simulink model "l64_dev"  (Simulink 7.9)
settings: Solver=ode45  StartTime=0.0  StopTime=525000  RelTol=1e-3
undefined symbols (not defined in the file): sfp
libraries: xbsIndex_r4 x835, xps_library x23, casper_library_delays x22, casper_library_misc x3
(part 3 of 8)

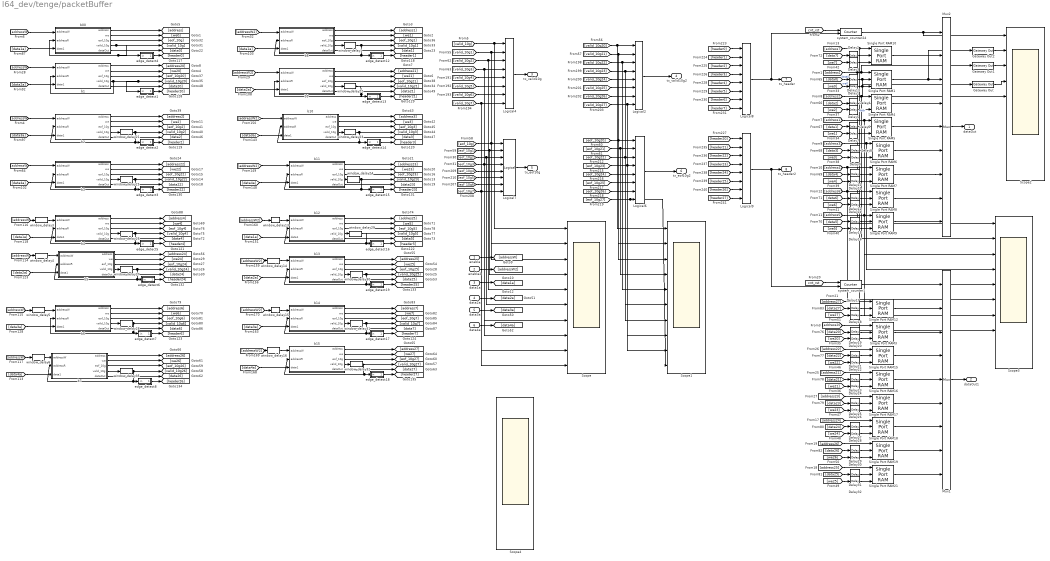
== system l64_dev/tenge/packetBuffer ==
  enable : Inport
  enable2 : Inport  Port=2
  data1a : Inport  Port=3
  data2a : Inport  Port=4
  data3a : Inport  Port=5
  data4a : Inport  Port=6
  Delay{1..32} (32 alike) : xbsIndex_r4/Delay  rst=off  infoeditControl=Selection of Reset will increase slice count due to use of real FFs and instead of SRLs  en=off  latency=2  dbl_ovrd=off  reg_retiming=on  block_type=delay
      settings: xl_area=[0, 0, 0, 0, 0, 0, 0]
  Gateway Out : xbsIndex_r4/Gateway Out  inherit_from_input=off  hdl_port=on  timing_constraint=None  locs_specified=off  LOCs={}  UseAsDAC=off  DACChannel='1'  block_type=gatewayout
  Gateway Out1 : xbsIndex_r4/Gateway Out  inherit_from_input=off  hdl_port=on  timing_constraint=None  locs_specified=off  LOCs={}  UseAsDAC=off  DACChannel='1'  block_type=gatewayout
  Gateway Out2 : xbsIndex_r4/Gateway Out  inherit_from_input=off  hdl_port=on  timing_constraint=None  locs_specified=off  LOCs={}  UseAsDAC=off  DACChannel='1'  block_type=gatewayout
  Logical{2,4,6..7} (4 alike) : xbsIndex_r4/Logical  logical_function=OR  inputs=8  en=off  latency=8  precision=Full  arith_type=Unsigned  n_bits=16  bin_pt=0  align_bp=on  dbl_ovrd=off  block_type=logical
      settings: block_version=11.4
  Logical8 : xbsIndex_r4/Logical  logical_function=OR  inputs=8  en=off  latency=4  precision=Full  arith_type=Unsigned  n_bits=16  bin_pt=0  align_bp=on  dbl_ovrd=off  block_type=logical
      settings: block_version=11.4
  Logical9 : xbsIndex_r4/Logical  logical_function=OR  inputs=8  en=off  latency=4  precision=Full  arith_type=Unsigned  n_bits=16  bin_pt=0  align_bp=on  dbl_ovrd=off  block_type=logical
      settings: block_version=11.4
  Mux1 : xbsIndex_r4/Mux  inputs=8  en=off  latency=2  precision=Full  arith_type="Signed  (2's comp)"  n_bits=8  bin_pt=2  quantization=Truncate  overflow=Wrap  dbl_ovrd=off  block_type=mux
      settings: xl_area=[0, 0, 0, 0, 0, 0, 0]
  Mux2 : xbsIndex_r4/Mux  inputs=8  en=off  latency=2  precision=Full  arith_type="Signed  (2's comp)"  n_bits=8  bin_pt=2  quantization=Truncate  overflow=Wrap  dbl_ovrd=off  block_type=mux
      settings: xl_area=[0, 0, 0, 0, 0, 0, 0]
  Scope{,1..4} (5 alike) : Scope  NumInputPorts=10
      Scope settings: YMin=0~0~0~4012~3800.95~-1~-5~-5~-5~-5  YMax=7000~1~1~4022~4201.05~1~5~5~5~5  SaveName=ScopeData3
      Scope1 settings: YMin=0~0~0~4012~3800.95~-1~-5~-5~-5~-5  YMax=7000~1~1~4022~4201.05~1~5~5~5~5  SaveName=ScopeData4
      Scope2 settings: YMin=0~0~0~4012~3800.95~-1~-5~-5~-5~-5  YMax=7000~1~1~4022~4201.05~1~5~5~5~5  SaveName=ScopeData5
      Scope3 settings: YMin=0~0~0~4012~3800.95~-1~-5~-5~-5~-5  YMax=7000~1~1~4022~4201.05~1~5~5~5~5  SaveName=ScopeData14
      Scope4 settings: YMin=0~0~0~4012~3800.95~-1~-5~-5~-5~-5  YMax=7000~1~1~4022~4201.05~1~5~5~5~5  SaveName=ScopeData16
  Single Port RAM{1,3..10,12,15..19,21} (16 alike) : xbsIndex_r4/Single Port RAM  depth=872  initVector=0  distributed_mem=Block RAM  write_mode=No Read On Write  rst=off  init_reg=0  en=off  latency=4  dbl_ovrd=off  optimize=Area  use_rpm=on  block_type=spram
  b00 : Subsystem
  b1 : Subsystem
  b10 : Subsystem
  b11 : Subsystem
  b12 : Subsystem
  b13 : Subsystem
  b14 : Subsystem
  b15 : Subsystem
  b2 : Subsystem
  b3 : Subsystem
  b4 : Subsystem
  b5 : Subsystem
  b6 : Subsystem
  b7 : Subsystem
  b8 : Subsystem
  b9 : Subsystem
  edge_detect1 : Subsystem  AncestorBlock=casper_library_misc/edge_detect  mask(edge_detect){edge=Rising, polarity=Active High, x_in=[0 0.08 0.08 0.16 0.16 0.24 0.24 0.32 0.32 0.4], y_in=[-1 -1  1  1  1  1  1  1  1  1], x_out=[0.6 0.68 0.68 0.76 0.76 0.84 0.84 0.92 0.92 1], y_out=[-1 -1  1  1 -1 -1 -1 -1 -1 -1]}
      mask prompts: edge "Edge Type"; polarity "Output Polarity"; x_in "Input X Positions"; y_in "Input Y Positions"; x_out "Output X Positions"; y_out "Output Y Positions"
      mask help: Output is active for one-cycle after each edge of the specified type (i.e. rising, falling or both).
      mask init: same as l64_dev/misc/edge_detect1
      settings: AttributesFormatString=|
      | rising edges
      | active high
      mask Help: Output is active for one-cycle after each edge of the specified type (i.e. rising, falling, or both).  Latency is zero.
      mask StyleString: popup(Rising|Falling|Both),popup(Active High|Active Low),edit,edit,edit,edit
      mask Display:
      | plot(x_in_num,0.5+y_in_num*0.2);
      | plot(x_out_num,0.5+y_out_num*0.2);
  edge_detect12 : Subsystem  AncestorBlock=casper_library_misc/edge_detect  mask(edge_detect){edge=Rising, polarity=Active High, x_in=[0 0.08 0.08 0.16 0.16 0.24 0.24 0.32 0.32 0.4], y_in=[-1 -1  1  1  1  1  1  1  1  1], x_out=[0.6 0.68 0.68 0.76 0.76 0.84 0.84 0.92 0.92 1], y_out=[-1 -1  1  1 -1 -1 -1 -1 -1 -1]}
      mask prompts: edge "Edge Type"; polarity "Output Polarity"; x_in "Input X Positions"; y_in "Input Y Positions"; x_out "Output X Positions"; y_out "Output Y Positions"
      mask help: Output is active for one-cycle after each edge of the specified type (i.e. rising, falling or both).
      mask init: same as l64_dev/misc/edge_detect1
      settings: AttributesFormatString=|
      | rising edges
      | active high
      mask Help: Output is active for one-cycle after each edge of the specified type (i.e. rising, falling, or both).  Latency is zero.
      mask StyleString: popup(Rising|Falling|Both),popup(Active High|Active Low),edit,edit,edit,edit
      mask Display:
      | plot(x_in_num,0.5+y_in_num*0.2);
      | plot(x_out_num,0.5+y_out_num*0.2);
  edge_detect13 : Subsystem  AncestorBlock=casper_library_misc/edge_detect  mask(edge_detect){edge=Rising, polarity=Active High, x_in=[0 0.08 0.08 0.16 0.16 0.24 0.24 0.32 0.32 0.4], y_in=[-1 -1  1  1  1  1  1  1  1  1], x_out=[0.6 0.68 0.68 0.76 0.76 0.84 0.84 0.92 0.92 1], y_out=[-1 -1  1  1 -1 -1 -1 -1 -1 -1]}
      mask prompts: edge "Edge Type"; polarity "Output Polarity"; x_in "Input X Positions"; y_in "Input Y Positions"; x_out "Output X Positions"; y_out "Output Y Positions"
      mask help: Output is active for one-cycle after each edge of the specified type (i.e. rising, falling or both).
      mask init: same as l64_dev/misc/edge_detect1
      settings: AttributesFormatString=|
      | rising edges
      | active high
      mask Help: Output is active for one-cycle after each edge of the specified type (i.e. rising, falling, or both).  Latency is zero.
      mask StyleString: popup(Rising|Falling|Both),popup(Active High|Active Low),edit,edit,edit,edit
      mask Display:
      | plot(x_in_num,0.5+y_in_num*0.2);
      | plot(x_out_num,0.5+y_out_num*0.2);
  edge_detect14 : Subsystem  AncestorBlock=casper_library_misc/edge_detect  mask(edge_detect){edge=Rising, polarity=Active High, x_in=[0 0.08 0.08 0.16 0.16 0.24 0.24 0.32 0.32 0.4], y_in=[-1 -1  1  1  1  1  1  1  1  1], x_out=[0.6 0.68 0.68 0.76 0.76 0.84 0.84 0.92 0.92 1], y_out=[-1 -1  1  1 -1 -1 -1 -1 -1 -1]}
      mask prompts: edge "Edge Type"; polarity "Output Polarity"; x_in "Input X Positions"; y_in "Input Y Positions"; x_out "Output X Positions"; y_out "Output Y Positions"
      mask help: Output is active for one-cycle after each edge of the specified type (i.e. rising, falling or both).
      mask init: same as l64_dev/misc/edge_detect1
      settings: AttributesFormatString=|
      | rising edges
      | active high
      mask Help: Output is active for one-cycle after each edge of the specified type (i.e. rising, falling, or both).  Latency is zero.
      mask StyleString: popup(Rising|Falling|Both),popup(Active High|Active Low),edit,edit,edit,edit
      mask Display:
      | plot(x_in_num,0.5+y_in_num*0.2);
      | plot(x_out_num,0.5+y_out_num*0.2);
  edge_detect15 : Subsystem  AncestorBlock=casper_library_misc/edge_detect  mask(edge_detect){edge=Rising, polarity=Active High, x_in=[0 0.08 0.08 0.16 0.16 0.24 0.24 0.32 0.32 0.4], y_in=[-1 -1  1  1  1  1  1  1  1  1], x_out=[0.6 0.68 0.68 0.76 0.76 0.84 0.84 0.92 0.92 1], y_out=[-1 -1  1  1 -1 -1 -1 -1 -1 -1]}
      mask prompts: edge "Edge Type"; polarity "Output Polarity"; x_in "Input X Positions"; y_in "Input Y Positions"; x_out "Output X Positions"; y_out "Output Y Positions"
      mask help: Output is active for one-cycle after each edge of the specified type (i.e. rising, falling or both).
      mask init: same as l64_dev/misc/edge_detect1
      settings: AttributesFormatString=|
      | rising edges
      | active high
      mask Help: Output is active for one-cycle after each edge of the specified type (i.e. rising, falling, or both).  Latency is zero.
      mask StyleString: popup(Rising|Falling|Both),popup(Active High|Active Low),edit,edit,edit,edit
      mask Display:
      | plot(x_in_num,0.5+y_in_num*0.2);
      | plot(x_out_num,0.5+y_out_num*0.2);
  edge_detect16 : Subsystem  AncestorBlock=casper_library_misc/edge_detect  mask(edge_detect){edge=Rising, polarity=Active High, x_in=[0 0.08 0.08 0.16 0.16 0.24 0.24 0.32 0.32 0.4], y_in=[-1 -1  1  1  1  1  1  1  1  1], x_out=[0.6 0.68 0.68 0.76 0.76 0.84 0.84 0.92 0.92 1], y_out=[-1 -1  1  1 -1 -1 -1 -1 -1 -1]}
      mask prompts: edge "Edge Type"; polarity "Output Polarity"; x_in "Input X Positions"; y_in "Input Y Positions"; x_out "Output X Positions"; y_out "Output Y Positions"
      mask help: Output is active for one-cycle after each edge of the specified type (i.e. rising, falling or both).
      mask init: same as l64_dev/misc/edge_detect1
      settings: AttributesFormatString=|
      | rising edges
      | active high
      mask Help: Output is active for one-cycle after each edge of the specified type (i.e. rising, falling, or both).  Latency is zero.
      mask StyleString: popup(Rising|Falling|Both),popup(Active High|Active Low),edit,edit,edit,edit
      mask Display:
      | plot(x_in_num,0.5+y_in_num*0.2);
      | plot(x_out_num,0.5+y_out_num*0.2);
  edge_detect17 : Subsystem  AncestorBlock=casper_library_misc/edge_detect  mask(edge_detect){edge=Rising, polarity=Active High, x_in=[0 0.08 0.08 0.16 0.16 0.24 0.24 0.32 0.32 0.4], y_in=[-1 -1  1  1  1  1  1  1  1  1], x_out=[0.6 0.68 0.68 0.76 0.76 0.84 0.84 0.92 0.92 1], y_out=[-1 -1  1  1 -1 -1 -1 -1 -1 -1]}
      mask prompts: edge "Edge Type"; polarity "Output Polarity"; x_in "Input X Positions"; y_in "Input Y Positions"; x_out "Output X Positions"; y_out "Output Y Positions"
      mask help: Output is active for one-cycle after each edge of the specified type (i.e. rising, falling or both).
      mask init: same as l64_dev/misc/edge_detect1
      settings: AttributesFormatString=|
      | rising edges
      | active high
      mask Help: Output is active for one-cycle after each edge of the specified type (i.e. rising, falling, or both).  Latency is zero.
      mask StyleString: popup(Rising|Falling|Both),popup(Active High|Active Low),edit,edit,edit,edit
      mask Display:
      | plot(x_in_num,0.5+y_in_num*0.2);
      | plot(x_out_num,0.5+y_out_num*0.2);
  edge_detect18 : Subsystem  AncestorBlock=casper_library_misc/edge_detect  mask(edge_detect){edge=Rising, polarity=Active High, x_in=[0 0.08 0.08 0.16 0.16 0.24 0.24 0.32 0.32 0.4], y_in=[-1 -1  1  1  1  1  1  1  1  1], x_out=[0.6 0.68 0.68 0.76 0.76 0.84 0.84 0.92 0.92 1], y_out=[-1 -1  1  1 -1 -1 -1 -1 -1 -1]}
      mask prompts: edge "Edge Type"; polarity "Output Polarity"; x_in "Input X Positions"; y_in "Input Y Positions"; x_out "Output X Positions"; y_out "Output Y Positions"
      mask help: Output is active for one-cycle after each edge of the specified type (i.e. rising, falling or both).
      mask init: same as l64_dev/misc/edge_detect1
      settings: AttributesFormatString=|
      | rising edges
      | active high
      mask Help: Output is active for one-cycle after each edge of the specified type (i.e. rising, falling, or both).  Latency is zero.
      mask StyleString: popup(Rising|Falling|Both),popup(Active High|Active Low),edit,edit,edit,edit
      mask Display:
      | plot(x_in_num,0.5+y_in_num*0.2);
      | plot(x_out_num,0.5+y_out_num*0.2);
  edge_detect19 : Subsystem  AncestorBlock=casper_library_misc/edge_detect  mask(edge_detect){edge=Rising, polarity=Active High, x_in=[0 0.08 0.08 0.16 0.16 0.24 0.24 0.32 0.32 0.4], y_in=[-1 -1  1  1  1  1  1  1  1  1], x_out=[0.6 0.68 0.68 0.76 0.76 0.84 0.84 0.92 0.92 1], y_out=[-1 -1  1  1 -1 -1 -1 -1 -1 -1]}
      mask prompts: edge "Edge Type"; polarity "Output Polarity"; x_in "Input X Positions"; y_in "Input Y Positions"; x_out "Output X Positions"; y_out "Output Y Positions"
      mask help: Output is active for one-cycle after each edge of the specified type (i.e. rising, falling or both).
      mask init: same as l64_dev/misc/edge_detect1
      settings: AttributesFormatString=|
      | rising edges
      | active high
      mask Help: Output is active for one-cycle after each edge of the specified type (i.e. rising, falling, or both).  Latency is zero.
      mask StyleString: popup(Rising|Falling|Both),popup(Active High|Active Low),edit,edit,edit,edit
      mask Display:
      | plot(x_in_num,0.5+y_in_num*0.2);
      | plot(x_out_num,0.5+y_out_num*0.2);
  edge_detect2 : Subsystem  AncestorBlock=casper_library_misc/edge_detect  mask(edge_detect){edge=Rising, polarity=Active High, x_in=[0 0.08 0.08 0.16 0.16 0.24 0.24 0.32 0.32 0.4], y_in=[-1 -1  1  1  1  1  1  1  1  1], x_out=[0.6 0.68 0.68 0.76 0.76 0.84 0.84 0.92 0.92 1], y_out=[-1 -1  1  1 -1 -1 -1 -1 -1 -1]}
      mask prompts: edge "Edge Type"; polarity "Output Polarity"; x_in "Input X Positions"; y_in "Input Y Positions"; x_out "Output X Positions"; y_out "Output Y Positions"
      mask help: Output is active for one-cycle after each edge of the specified type (i.e. rising, falling or both).
      mask init: same as l64_dev/misc/edge_detect1
      settings: AttributesFormatString=|
      | rising edges
      | active high
      mask Help: Output is active for one-cycle after each edge of the specified type (i.e. rising, falling, or both).  Latency is zero.
      mask StyleString: popup(Rising|Falling|Both),popup(Active High|Active Low),edit,edit,edit,edit
      mask Display:
      | plot(x_in_num,0.5+y_in_num*0.2);
      | plot(x_out_num,0.5+y_out_num*0.2);
  edge_detect3 : Subsystem  AncestorBlock=casper_library_misc/edge_detect  mask(edge_detect){edge=Rising, polarity=Active High, x_in=[0 0.08 0.08 0.16 0.16 0.24 0.24 0.32 0.32 0.4], y_in=[-1 -1  1  1  1  1  1  1  1  1], x_out=[0.6 0.68 0.68 0.76 0.76 0.84 0.84 0.92 0.92 1], y_out=[-1 -1  1  1 -1 -1 -1 -1 -1 -1]}
      mask prompts: edge "Edge Type"; polarity "Output Polarity"; x_in "Input X Positions"; y_in "Input Y Positions"; x_out "Output X Positions"; y_out "Output Y Positions"
      mask help: Output is active for one-cycle after each edge of the specified type (i.e. rising, falling or both).
      mask init: same as l64_dev/misc/edge_detect1
      settings: AttributesFormatString=|
      | rising edges
      | active high
      mask Help: Output is active for one-cycle after each edge of the specified type (i.e. rising, falling, or both).  Latency is zero.
      mask StyleString: popup(Rising|Falling|Both),popup(Active High|Active Low),edit,edit,edit,edit
      mask Display:
      | plot(x_in_num,0.5+y_in_num*0.2);
      | plot(x_out_num,0.5+y_out_num*0.2);
  edge_detect4 : Subsystem  AncestorBlock=casper_library_misc/edge_detect  mask(edge_detect){edge=Rising, polarity=Active High, x_in=[0 0.08 0.08 0.16 0.16 0.24 0.24 0.32 0.32 0.4], y_in=[-1 -1  1  1  1  1  1  1  1  1], x_out=[0.6 0.68 0.68 0.76 0.76 0.84 0.84 0.92 0.92 1], y_out=[-1 -1  1  1 -1 -1 -1 -1 -1 -1]}
      mask prompts: edge "Edge Type"; polarity "Output Polarity"; x_in "Input X Positions"; y_in "Input Y Positions"; x_out "Output X Positions"; y_out "Output Y Positions"
      mask help: Output is active for one-cycle after each edge of the specified type (i.e. rising, falling or both).
      mask init: same as l64_dev/misc/edge_detect1
      settings: AttributesFormatString=|
      | rising edges
      | active high
      mask Help: Output is active for one-cycle after each edge of the specified type (i.e. rising, falling, or both).  Latency is zero.
      mask StyleString: popup(Rising|Falling|Both),popup(Active High|Active Low),edit,edit,edit,edit
      mask Display:
      | plot(x_in_num,0.5+y_in_num*0.2);
      | plot(x_out_num,0.5+y_out_num*0.2);
  edge_detect5 : Subsystem  AncestorBlock=casper_library_misc/edge_detect  mask(edge_detect){edge=Rising, polarity=Active High, x_in=[0 0.08 0.08 0.16 0.16 0.24 0.24 0.32 0.32 0.4], y_in=[-1 -1  1  1  1  1  1  1  1  1], x_out=[0.6 0.68 0.68 0.76 0.76 0.84 0.84 0.92 0.92 1], y_out=[-1 -1  1  1 -1 -1 -1 -1 -1 -1]}
      mask prompts: edge "Edge Type"; polarity "Output Polarity"; x_in "Input X Positions"; y_in "Input Y Positions"; x_out "Output X Positions"; y_out "Output Y Positions"
      mask help: Output is active for one-cycle after each edge of the specified type (i.e. rising, falling or both).
      mask init: same as l64_dev/misc/edge_detect1
      settings: AttributesFormatString=|
      | rising edges
      | active high
      mask Help: Output is active for one-cycle after each edge of the specified type (i.e. rising, falling, or both).  Latency is zero.
      mask StyleString: popup(Rising|Falling|Both),popup(Active High|Active Low),edit,edit,edit,edit
      mask Display:
      | plot(x_in_num,0.5+y_in_num*0.2);
      | plot(x_out_num,0.5+y_out_num*0.2);
  edge_detect6 : Subsystem  AncestorBlock=casper_library_misc/edge_detect  mask(edge_detect){edge=Rising, polarity=Active High, x_in=[0 0.08 0.08 0.16 0.16 0.24 0.24 0.32 0.32 0.4], y_in=[-1 -1  1  1  1  1  1  1  1  1], x_out=[0.6 0.68 0.68 0.76 0.76 0.84 0.84 0.92 0.92 1], y_out=[-1 -1  1  1 -1 -1 -1 -1 -1 -1]}
      mask prompts: edge "Edge Type"; polarity "Output Polarity"; x_in "Input X Positions"; y_in "Input Y Positions"; x_out "Output X Positions"; y_out "Output Y Positions"
      mask help: Output is active for one-cycle after each edge of the specified type (i.e. rising, falling or both).
      mask init: same as l64_dev/misc/edge_detect1
      settings: AttributesFormatString=|
      | rising edges
      | active high
      mask Help: Output is active for one-cycle after each edge of the specified type (i.e. rising, falling, or both).  Latency is zero.
      mask StyleString: popup(Rising|Falling|Both),popup(Active High|Active Low),edit,edit,edit,edit
      mask Display:
      | plot(x_in_num,0.5+y_in_num*0.2);
      | plot(x_out_num,0.5+y_out_num*0.2);
  edge_detect7 : Subsystem  AncestorBlock=casper_library_misc/edge_detect  mask(edge_detect){edge=Rising, polarity=Active High, x_in=[0 0.08 0.08 0.16 0.16 0.24 0.24 0.32 0.32 0.4], y_in=[-1 -1  1  1  1  1  1  1  1  1], x_out=[0.6 0.68 0.68 0.76 0.76 0.84 0.84 0.92 0.92 1], y_out=[-1 -1  1  1 -1 -1 -1 -1 -1 -1]}
      mask prompts: edge "Edge Type"; polarity "Output Polarity"; x_in "Input X Positions"; y_in "Input Y Positions"; x_out "Output X Positions"; y_out "Output Y Positions"
      mask help: Output is active for one-cycle after each edge of the specified type (i.e. rising, falling or both).
      mask init: same as l64_dev/misc/edge_detect1
      settings: AttributesFormatString=|
      | rising edges
      | active high
      mask Help: Output is active for one-cycle after each edge of the specified type (i.e. rising, falling, or both).  Latency is zero.
      mask StyleString: popup(Rising|Falling|Both),popup(Active High|Active Low),edit,edit,edit,edit
      mask Display:
      | plot(x_in_num,0.5+y_in_num*0.2);
      | plot(x_out_num,0.5+y_out_num*0.2);
  edge_detect8 : Subsystem  AncestorBlock=casper_library_misc/edge_detect  mask(edge_detect){edge=Rising, polarity=Active High, x_in=[0 0.08 0.08 0.16 0.16 0.24 0.24 0.32 0.32 0.4], y_in=[-1 -1  1  1  1  1  1  1  1  1], x_out=[0.6 0.68 0.68 0.76 0.76 0.84 0.84 0.92 0.92 1], y_out=[-1 -1  1  1 -1 -1 -1 -1 -1 -1]}
      mask prompts: edge "Edge Type"; polarity "Output Polarity"; x_in "Input X Positions"; y_in "Input Y Positions"; x_out "Output X Positions"; y_out "Output Y Positions"
      mask help: Output is active for one-cycle after each edge of the specified type (i.e. rising, falling or both).
      mask init: same as l64_dev/misc/edge_detect1
      settings: AttributesFormatString=|
      | rising edges
      | active high
      mask Help: Output is active for one-cycle after each edge of the specified type (i.e. rising, falling, or both).  Latency is zero.
      mask StyleString: popup(Rising|Falling|Both),popup(Active High|Active Low),edit,edit,edit,edit
      mask Display:
      | plot(x_in_num,0.5+y_in_num*0.2);
      | plot(x_out_num,0.5+y_out_num*0.2);
  system_counter1 : xbsIndex_r4/Counter  cnt_type=Free Running  cnt_to=7  operation=Up  start_count=0  cnt_by_val=1  arith_type=Unsigned  n_bits=3  bin_pt=0  load_pin=off  rst=on  en=on  explicit_period=on  period=1  dbl_ovrd=off  use_behavioral_HDL=off  implementation=Fabric  block_type=counter
      settings: block_version=11.4
  system_counter24 : xbsIndex_r4/Counter  cnt_type=Free Running  cnt_to=7  operation=Up  start_count=0  cnt_by_val=1  arith_type=Unsigned  n_bits=3  bin_pt=0  load_pin=off  rst=on  en=on  explicit_period=on  period=1  dbl_ovrd=off  use_behavioral_HDL=off  implementation=Fabric  block_type=counter
      settings: block_version=11.4
  window_delay1 : casper_library_delays/window_delay  delay=1400
  window_delay{3..6,13..16} (8 alike) : casper_library_delays/window_delay  delay=1200
  window_delay21 : casper_library_delays/window_delay  delay=700
  window_delay22 : casper_library_delays/window_delay  delay=1400
  window_delay23 : casper_library_delays/window_delay  delay=2100
  window_delay24 : casper_library_delays/window_delay  delay=2100
  window_delay25 : casper_library_delays/window_delay  delay=700
  window_delay26 : casper_library_delays/window_delay  delay=2800
  window_delay27 : casper_library_delays/window_delay  delay=2800
  window_delay28 : casper_library_delays/window_delay  delay=3500
  window_delay29 : casper_library_delays/window_delay  delay=4200
  window_delay30 : casper_library_delays/window_delay  delay=4200
  window_delay31 : casper_library_delays/window_delay  delay=4900
  window_delay32 : casper_library_delays/window_delay  delay=4900
  window_delay35 : casper_library_delays/window_delay  delay=3500
  dataOut : Outport
  dataOut1 : Outport  Port=2
  tx_valid10g : Outport  Port=3
  tx_valid10g2 : Outport  Port=4
  tx_eof10g : Outport  Port=5
  tx_eof10g2 : Outport  Port=6
  tx_header : Outport  Port=7
  tx_header2 : Outport  Port=8
  wires:
  Single Port RAM1/1 -> Mux2/3, Gateway Out2/1
  Single Port RAM4/1 -> Mux2/4
  Single Port RAM5/1 -> Mux2/5
  Single Port RAM6/1 -> Mux2/6
  Single Port RAM7/1 -> Mux2/7
  Single Port RAM8/1 -> Mux2/8
  Mux2/1 -> dataOut/1
  Single Port RAM3/1 -> Mux1/3
  Single Port RAM15/1 -> Mux1/4
  Single Port RAM16/1 -> Mux1/5
  Single Port RAM17/1 -> Mux1/6
  Single Port RAM18/1 -> Mux1/7
  Single Port RAM19/1 -> Mux1/8
  Single Port RAM21/1 -> Mux1/9
  Mux1/1 -> dataOut1/1
  ? -> ?
  enable/1 -> [addressW]
  enable2/1 -> [addressW2]
  [addressW] -> b00/1(addressW)
  b00/1(address) -> [address]
  b00/2(we) -> [we0]
  [addressW] -> b1/1(addressW)
  b1/1(address) -> [address20]
  b1/2(we) -> [we20]
  b8/1(address) -> [address1]
  [addressW2] -> b9/1(addressW)
  b00/4(valid_10g) -> [valid_10g], edge_detect4/1(in), b00/2(addressR)
  [valid_10g] -> Logical4/1, Scope/1
  [valid_10g1] -> Logical4/2, Scope/3
  Logical4/1 -> tx_valid10g/1
  [valid_10g20] -> Logical2/1, Scope1/1
  [valid_10g21] -> Logical2/2, Scope1/3
  Logical2/1 -> tx_valid10g2/1
  b00/3(eof_10g) -> [eof_10g]
  [eof_10g] -> Logical7/1, Scope/2
  [eof_10g1] -> Logical7/2, Scope/4
  Logical7/1 -> tx_eof10g/1
  [eof_10g20] -> Logical6/1, Scope1/2
  [eof_10g21] -> Logical6/2, Scope1/4
  Logical6/1 -> tx_eof10g2/1
  b8/2(we) -> [we1]
  b1/4(valid_10g) -> b1/2(addressR), edge_detect1/1(in), [valid_10g20]
  b1/3(eof_10g) -> [eof_10g20]
  b8/3(eof_10g) -> [eof_10g1]
  [addressW] -> b2/1(addressW)
  b2/1(address) -> [address2]
  b2/2(we) -> [we2]
  b2/4(valid_10g) -> window_delay21/1
  b2/3(eof_10g) -> [eof_10g2]
  [eof_10g2] -> Logical7/3, Scope/6
  [eof_10g3] -> Logical7/4, Scope/8
  [valid_10g2] -> Logical4/3, Scope/5
  [valid_10g3] -> Logical4/4, Scope/7
  [addressW] -> b3/1(addressW)
  [addressW2] -> b8/1(addressW)
  b00/5(dataOut) -> [data0]
  b1/5(dataOut) -> [data20]
  b2/5(dataOut) -> [data2]
  b8/5(dataOut) -> [data1]
  data1a/1 -> [data1a]
  data2a/1 -> [data2a]
  data3a/1 -> [data3a]
  data4a/1 -> [data4a]
  [data1a] -> b00/3(data1)
  [data3a] -> b2/3(data1)
  [data4a] -> b3/3(data1)
  [addressW] -> window_delay3/1
  [addressW] -> window_delay4/1
  [addressW] -> window_delay5/1
  b6/1(address) -> [address6]
  b6/2(we) -> [we6]
  b6/4(valid_10g) -> window_delay28/1
  b6/3(eof_10g) -> [eof_10g6]
  [addressW] -> window_delay6/1
  window_delay4/1 -> b5/1(addressW)
  b6/5(dataOut) -> [data6]
  [data4a] -> b7/3(data1)
  [addressW2] -> b11/1(addressW)
  [data3a] -> b10/3(data1)
  [data4a] -> b11/3(data1)
  [addressW2] -> window_delay14/1
  window_delay14/1 -> b13/1(addressW)
  [addressW2] -> window_delay13/1
  [addressW2] -> window_delay16/1
  window_delay16/1 -> b15/1(addressW)
  [addressW2] -> window_delay15/1
  [data3a] -> b14/3(data1)
  [data4a] -> b15/3(data1)
  [valid_10g4] -> Logical4/5
  [valid_10g5] -> Logical4/6
  [valid_10g6] -> Logical4/7
  [valid_10g7] -> Logical4/8, Scope/9
  [valid_10g22] -> Logical2/3, Scope1/5
  [valid_10g23] -> Logical2/4, Scope1/7
  [valid_10g24] -> Logical2/5
  [valid_10g25] -> Logical2/6
  [valid_10g26] -> Logical2/7
  [valid_10g27] -> Logical2/8, Scope1/9
  [eof_10g4] -> Logical7/5
  [eof_10g5] -> Logical7/6
  [eof_10g6] -> Logical7/7
  [eof_10g7] -> Logical7/8, Scope/10
  [eof_10g22] -> Logical6/3, Scope1/6
  [eof_10g23] -> Logical6/4, Scope1/8
  [eof_10g24] -> Logical6/5
  [eof_10g25] -> Logical6/6
  [eof_10g26] -> Logical6/7
  [eof_10g27] -> Logical6/8, Scope1/10
  [header0] -> Logical8/1
  [header1] -> Logical8/2
  [header2] -> Logical8/3
  [header3] -> Logical8/4
  [header4] -> Logical8/5
  [header5] -> Logical8/6
  [header6] -> Logical8/7
  [header7] -> Logical8/8
  Logical8/1 -> tx_header/1, system_counter24/2
  [header20] -> Logical9/1
  [header21] -> Logical9/2
  [header22] -> Logical9/3
  [header23] -> Logical9/4
  [header24] -> Logical9/5
  [header25] -> Logical9/6
  [header26] -> Logical9/7
  [header27] -> Logical9/8
  Logical9/1 -> tx_header2/1, system_counter1/2
  edge_detect4/1(out) -> [header0]
  window_delay3/1 -> b4/1(addressW)
  window_delay5/1 -> b6/1(addressW)
  window_delay6/1 -> b7/1(addressW)
  window_delay13/1 -> b12/1(addressW)
  window_delay15/1 -> b14/1(addressW)
  edge_detect1/1(out) -> [header20]
  edge_detect7/1(out) -> [header6]
  edge_detect12/1(out) -> [header1]
  system_counter24/1 -> Mux2/1, Scope2/1
  system_counter1/1 -> Mux1/1
  [cnt_rst] -> system_counter24/1
  [cnt_rst] -> system_counter1/1
  window_delay21/1 -> [valid_10g2], edge_detect2/1(in), b2/2(addressR)
  edge_detect2/1(out) -> [header2]
  b3/1(address) -> [address22]
  b3/2(we) -> [we22]
  b3/5(dataOut) -> [data22]
  window_delay25/1 -> [valid_10g22], edge_detect3/1(in), b3/2(addressR)
  b3/3(eof_10g) -> [eof_10g22]
  b3/4(valid_10g) -> window_delay25/1
  edge_detect3/1(out) -> [header22]
  b4/5(dataOut) -> [data4]
  window_delay26/1 -> [valid_10g4], edge_detect5/1(in), b4/2(addressR)
  b4/3(eof_10g) -> [eof_10g4]
  b4/4(valid_10g) -> window_delay26/1
  edge_detect5/1(out) -> [header4]
  b4/1(address) -> [address4]
  b4/2(we) -> [we4]
  b5/1(address) -> [address24]
  b5/2(we) -> [we24]
  b5/5(dataOut) -> [data24]
  window_delay27/1 -> [valid_10g24], edge_detect6/1(in), b5/2(addressR)
  b5/3(eof_10g) -> [eof_10g24]
  b5/4(valid_10g) -> window_delay27/1
  edge_detect6/1(out) -> [header24]
  b7/1(address) -> [address26]
  b7/2(we) -> [we26]
  b7/5(dataOut) -> [data26]
  window_delay35/1 -> [valid_10g26], edge_detect8/1(in), b7/2(addressR)
  b7/3(eof_10g) -> [eof_10g26]
  b7/4(valid_10g) -> window_delay35/1
  edge_detect8/1(out) -> [header26]
  window_delay22/1 -> [valid_10g21], edge_detect13/1(in), b9/2(addressR)
  edge_detect13/1(out) -> [header21]
  b10/1(address) -> [address3]
  b10/2(we) -> [we3]
  b10/5(dataOut) -> [data3]
  edge_detect14/1(out) -> [header3]
  b10/3(eof_10g) -> [eof_10g3]
  b10/4(valid_10g) -> window_delay23/1
  b11/1(address) -> [address23]
  b11/2(we) -> [we23]
  b11/5(dataOut) -> [data23]
  edge_detect15/1(out) -> [header23]
  b11/3(eof_10g) -> [eof_10g23]
  b11/4(valid_10g) -> window_delay24/1
  b12/1(address) -> [address5]
  b12/2(we) -> [we5]
  b12/5(dataOut) -> [data5]
  window_delay29/1 -> [valid_10g5], edge_detect16/1(in), b12/2(addressR)
  edge_detect16/1(out) -> [header5]
  b14/1(address) -> [address7]
  b14/2(we) -> [we7]
  b14/5(dataOut) -> [data7]
  window_delay31/1 -> [valid_10g7], edge_detect17/1(in), b14/2(addressR)
  edge_detect17/1(out) -> [header7]
  b15/1(address) -> [address27]
  b15/2(we) -> [we27]
  b15/5(dataOut) -> [data27]
  window_delay32/1 -> [valid_10g27], edge_detect18/1(in), b15/2(addressR)
  edge_detect18/1(out) -> [header27]
  b13/1(address) -> [address25]
  b13/2(we) -> [we25]
  b13/5(dataOut) -> [data25]
  window_delay30/1 -> [valid_10g25], edge_detect19/1(in), b13/2(addressR)
  edge_detect19/1(out) -> [header25]
  b12/3(eof_10g) -> [eof_10g5]
  b12/4(valid_10g) -> window_delay29/1
  b13/4(valid_10g) -> window_delay30/1
  b13/3(eof_10g) -> [eof_10g25]
  b14/3(eof_10g) -> [eof_10g7]
  b14/4(valid_10g) -> window_delay31/1
  b15/3(eof_10g) -> [eof_10g27]
  b15/4(valid_10g) -> window_delay32/1
  window_delay28/1 -> [valid_10g6], edge_detect7/1(in), b6/2(addressR)
  [address] -> Single Port RAM1/1, Gateway Out1/1, Scope3/1  "addr"
  [address2] -> Single Port RAM4/1, Scope3/2
  [address1] -> Single Port RAM5/1, Scope3/3
  [address3] -> Single Port RAM6/1, Scope3/4
  [address4] -> Single Port RAM7/1, Scope3/5
  [address6] -> Single Port RAM8/1, Scope3/6
  [address5] -> Single Port RAM9/1, Scope3/7
  [we0] -> Delay1/1  "we0"
  [we2] -> Delay5/1
  [we1] -> Delay7/1
  [we3] -> Delay9/1
  [we4] -> Delay11/1
  [we6] -> Delay14/1
  [we5] -> Delay16/1
  [data0] -> Delay13/1  "data0"
  [data2] -> Delay4/1
  [data1] -> Delay6/1
  [data3] -> Delay8/1
  [data4] -> Delay10/1
  [data6] -> Delay12/1
  [data5] -> Delay15/1
  [address20] -> Single Port RAM3/1
  [address22] -> Single Port RAM15/1
  [address23] -> Single Port RAM17/1
  [address24] -> Single Port RAM18/1
  [address26] -> Single Port RAM19/1
  [address25] -> Single Port RAM21/1
  [address21] -> Single Port RAM16/1
  [we20] -> Delay20/1
  [we22] -> Delay22/1
  [we21] -> Delay24/1
  [we23] -> Delay26/1
  [we24] -> Delay28/1
  [we26] -> Delay30/1
  [we25] -> Delay32/1
  [data20] -> Delay19/1
  [data22] -> Delay21/1
  [data21] -> Delay23/1
  [data23] -> Delay25/1
  [data24] -> Delay27/1
  [data26] -> Delay29/1
  [data25] -> Delay31/1
  Single Port RAM10/1 -> Mux2/2
  [address7] -> Single Port RAM10/1, Scope3/8
  [we7] -> Delay3/1
  [data7] -> Delay2/1
  Single Port RAM12/1 -> Mux1/2
  [address27] -> Single Port RAM12/1
  [we27] -> Delay18/1
  [data27] -> Delay17/1
  [addressW2] -> b10/1(addressW)
  b9/5(dataOut) -> [data21]
  b9/4(valid_10g) -> window_delay22/1
  b9/3(eof_10g) -> [eof_10g21]
  b9/2(we) -> [we21]
  b9/1(address) -> [address21]
  [data1a] -> b4/3(data1)
  [data2a] -> b1/3(data1)
  [data2a] -> b5/3(data1)
  [data3a] -> b6/3(data1)
  [data2a] -> b9/3(data1)
  [data1a] -> b12/3(data1)
  [data2a] -> b13/3(data1)
  Single Port RAM9/1 -> Mux2/9
  [data1a] -> b8/3(data1)
  b8/4(valid_10g) -> window_delay1/1
  window_delay1/1 -> [valid_10g1], edge_detect12/1(in), b8/2(addressR)
  window_delay23/1 -> [valid_10g3], edge_detect14/1(in), b10/2(addressR)
  window_delay24/1 -> [valid_10g23], edge_detect15/1(in), b11/2(addressR)
  Gateway Out/1 -> Scope2/4
  Delay13/1 -> Single Port RAM1/2, Gateway Out/1
  Delay1/1 -> Single Port RAM1/3, Scope2/5
  Delay2/1 -> Single Port RAM10/2
  Delay4/1 -> Single Port RAM4/2
  Delay5/1 -> Single Port RAM4/3
  Delay6/1 -> Single Port RAM5/2
  Delay8/1 -> Single Port RAM6/2
  Delay9/1 -> Single Port RAM6/3
  Delay7/1 -> Single Port RAM5/3
  Delay10/1 -> Single Port RAM7/2
  Delay11/1 -> Single Port RAM7/3
  Delay12/1 -> Single Port RAM8/2
  Delay14/1 -> Single Port RAM8/3
  Delay15/1 -> Single Port RAM9/2
  Delay16/1 -> Single Port RAM9/3
  Delay17/1 -> Single Port RAM12/2
  Delay18/1 -> Single Port RAM12/3
  Delay19/1 -> Single Port RAM3/2
  Delay20/1 -> Single Port RAM3/3
  Delay21/1 -> Single Port RAM15/2
  Delay22/1 -> Single Port RAM15/3
  Delay23/1 -> Single Port RAM16/2
  Delay24/1 -> Single Port RAM16/3
  Delay25/1 -> Single Port RAM17/2
  Delay26/1 -> Single Port RAM17/3
  Delay27/1 -> Single Port RAM18/2
  Delay28/1 -> Single Port RAM18/3
  Delay29/1 -> Single Port RAM19/2
  Delay30/1 -> Single Port RAM19/3
  Delay31/1 -> Single Port RAM21/2
  Delay32/1 -> Single Port RAM21/3
  Delay3/1 -> Single Port RAM10/3
  Gateway Out1/1 -> Scope2/3
  Gateway Out2/1 -> Scope2/2

== system l64_dev/fft/sync_gen/rst_gen ==
  arm : Inport
  sync_in : Inport  Port=2
  Constant : xbsIndex_r4/Constant  const=0  gui_display_data_type=Fixed-point  arith_type=Unsigned  n_bits=ceil(log2(reset_period+1))+1  bin_pt=0  preci_type=Single  exp_width=8  frac_width=24  explicit_period=off  period=1  equ=P=C  opselect=C  inp2=PCIN>>17  opr=+  inp1=P  carry=CIN  dbl_ovrd=off  block_type=constant
  Counter : xbsIndex_r4/Counter  cnt_type=Free Running  cnt_to=0  operation=Down  start_count=reset_period+1  cnt_by_val=1  arith_type=Unsigned  n_bits=ceil(log2(reset_period+1))+1  bin_pt=0  load_pin=off  rst=on  en=on  explicit_period=on  period=1  dbl_ovrd=off  use_behavioral_HDL=off  implementation=Fabric  use_rpm=off  block_type=counter
  Logical : xbsIndex_r4/Logical  logical_function=AND  inputs=2  en=off  latency=0  precision=Full  arith_type=Unsigned  n_bits=16  bin_pt=0  align_bp=on  dbl_ovrd=off  block_type=logical
  Relational : xbsIndex_r4/Relational  mode=a>b  en=off  latency=0  dbl_ovrd=off  block_type=relational
      settings: block_version=10.1.3
  mrst : Outport
  wires:
  arm/1 -> Counter/1
  Counter/1 -> Relational/1
  Constant/1 -> Relational/2
  sync_in/1 -> Logical/1
  Relational/1 -> mrst/1, Logical/2
  Logical/1 -> Counter/2

== system l64_dev/fft/sync_gen/sync_gen ==
  rst : Inport
  sync_period : Inport  Port=2
  Delay : xbsIndex_r4/Delay  rst=off  infoeditControl=Selection of Reset will increase slice count due to use of real FFs and instead of SRLs  en=off  latency=1  dbl_ovrd=off  reg_retiming=off  block_type=delay
  Logical : xbsIndex_r4/Logical  logical_function=OR  inputs=2  en=off  latency=1  precision=Full  arith_type=Unsigned  n_bits=16  bin_pt=0  align_bp=on  dbl_ovrd=off  block_type=logical
  Logical1 : xbsIndex_r4/Logical  logical_function=OR  inputs=2  en=off  latency=0  precision=Full  arith_type=Unsigned  n_bits=16  bin_pt=0  align_bp=on  dbl_ovrd=off  block_type=logical
  Relational : xbsIndex_r4/Relational  mode=a>=b  en=off  latency=1  dbl_ovrd=off  block_type=relational
      settings: block_version=10.1.3
  negedge : casper_library_misc/negedge  Tag=Rising Edge Detector
  posedge1 : casper_library_misc/posedge  Tag=Rising Edge Detector
  sync_count : xbsIndex_r4/Counter  cnt_type=Free Running  cnt_to=Inf  operation=Up  start_count=3  cnt_by_val=1  arith_type=Unsigned  n_bits=sync_gen_bits  bin_pt=0  load_pin=off  rst=on  en=off  explicit_period=on  period=1  dbl_ovrd=off  use_behavioral_HDL=on  implementation=Fabric  use_rpm=on  block_type=counter
  sync : Outport
  wires:
  Delay/1 -> Logical/1
  posedge1/1 -> Logical1/2, Logical/2
  sync_period/1 -> Relational/2
  Logical1/1 -> sync/1
  rst/1 -> Delay/1, negedge/1
  negedge/1 -> Logical1/1
  Logical/1 -> sync_count/1
  Relational/1 -> posedge1/1
  sync_count/1 -> Relational/1

== system l64_dev/tenge/chSel/edge_detect2 ==
  in : Inport
  Delay : xbsIndex_r4/Delay  rst=off  infoeditControl=Selection of Reset will increase slice count due to use of real FFs and instead of SRLs  en=off  latency=1  dbl_ovrd=off  reg_retiming=off  block_type=delay
      settings: xl_area=[0, 0, 0, 0, 0, 0, 0]
  Inverter : xbsIndex_r4/Inverter  en=off  latency=0  dbl_ovrd=off  block_type=inv
      settings: xl_area=[0, 0, 0, 0, 0, 0, 0]
  edge_op : xbsIndex_r4/Logical  logical_function=AND  inputs=2  en=off  latency=0  precision=Full  arith_type=Unsigned  n_bits=8  bin_pt=2  align_bp=on  dbl_ovrd=off  block_type=logical
      settings: xl_area=[0, 0, 0, 0, 0, 0, 0]
  out : Outport
  wires:
  Inverter/1 -> edge_op/1
  edge_op/1 -> out/1
  in/1 -> Inverter/1, Delay/1
  Delay/1 -> edge_op/2

== system l64_dev/tenge/chSel/edge_detect3 ==
  in : Inport
  Delay : xbsIndex_r4/Delay  rst=off  infoeditControl=Selection of Reset will increase slice count due to use of real FFs and instead of SRLs  en=off  latency=1  dbl_ovrd=off  reg_retiming=off  block_type=delay
      settings: xl_area=[0, 0, 0, 0, 0, 0, 0]
  Inverter : xbsIndex_r4/Inverter  en=off  latency=0  dbl_ovrd=off  block_type=inv
      settings: xl_area=[0, 0, 0, 0, 0, 0, 0]
  edge_op : xbsIndex_r4/Logical  logical_function=NOR  inputs=2  en=off  latency=0  precision=Full  arith_type=Unsigned  n_bits=8  bin_pt=2  align_bp=on  dbl_ovrd=off  block_type=logical
      settings: xl_area=[0, 0, 0, 0, 0, 0, 0]
  out : Outport
  wires:
  Inverter/1 -> edge_op/1
  edge_op/1 -> out/1
  in/1 -> Inverter/1, Delay/1
  Delay/1 -> edge_op/2

== system l64_dev/tenge/chSel/edge_detect4 ==
  in : Inport
  Delay : xbsIndex_r4/Delay  rst=off  infoeditControl=Selection of Reset will increase slice count due to use of real FFs and instead of SRLs  en=off  latency=1  dbl_ovrd=off  reg_retiming=off  block_type=delay
      settings: xl_area=[0, 0, 0, 0, 0, 0, 0]
  Inverter : xbsIndex_r4/Inverter  en=off  latency=0  dbl_ovrd=off  block_type=inv
      settings: xl_area=[0, 0, 0, 0, 0, 0, 0]
  edge_op : xbsIndex_r4/Logical  logical_function=AND  inputs=2  en=off  latency=0  precision=Full  arith_type=Unsigned  n_bits=8  bin_pt=2  align_bp=on  dbl_ovrd=off  block_type=logical
      settings: xl_area=[0, 0, 0, 0, 0, 0, 0]
  out : Outport
  wires:
  Inverter/1 -> edge_op/1
  edge_op/1 -> out/1
  in/1 -> Inverter/1, Delay/1
  Delay/1 -> edge_op/2

== system l64_dev/tenge/chSel/edge_detect5 ==
  in : Inport
  Delay : xbsIndex_r4/Delay  rst=off  infoeditControl=Selection of Reset will increase slice count due to use of real FFs and instead of SRLs  en=off  latency=1  dbl_ovrd=off  reg_retiming=off  block_type=delay
      settings: xl_area=[0, 0, 0, 0, 0, 0, 0]
  Inverter : xbsIndex_r4/Inverter  en=off  latency=0  dbl_ovrd=off  block_type=inv
      settings: xl_area=[0, 0, 0, 0, 0, 0, 0]
  edge_op : xbsIndex_r4/Logical  logical_function=AND  inputs=2  en=off  latency=0  precision=Full  arith_type=Unsigned  n_bits=8  bin_pt=2  align_bp=on  dbl_ovrd=off  block_type=logical
      settings: xl_area=[0, 0, 0, 0, 0, 0, 0]
  out : Outport
  wires:
  Inverter/1 -> edge_op/1
  edge_op/1 -> out/1
  in/1 -> Inverter/1, Delay/1
  Delay/1 -> edge_op/2

== system l64_dev/tenge/chSel/edge_detect7 ==
  in : Inport
  Delay : xbsIndex_r4/Delay  rst=off  infoeditControl=Selection of Reset will increase slice count due to use of real FFs and instead of SRLs  en=off  latency=1  dbl_ovrd=off  reg_retiming=off  block_type=delay
      settings: xl_area=[0, 0, 0, 0, 0, 0, 0]
  Inverter : xbsIndex_r4/Inverter  en=off  latency=0  dbl_ovrd=off  block_type=inv
      settings: xl_area=[0, 0, 0, 0, 0, 0, 0]
  edge_op : xbsIndex_r4/Logical  logical_function=NOR  inputs=2  en=off  latency=0  precision=Full  arith_type=Unsigned  n_bits=8  bin_pt=2  align_bp=on  dbl_ovrd=off  block_type=logical
      settings: xl_area=[0, 0, 0, 0, 0, 0, 0]
  out : Outport
  wires:
  Inverter/1 -> edge_op/1
  edge_op/1 -> out/1
  in/1 -> Inverter/1, Delay/1
  Delay/1 -> edge_op/2

== system l64_dev/tenge/header/edge_detect1 ==
  in : Inport
  Delay : xbsIndex_r4/Delay  rst=off  infoeditControl=Selection of Reset will increase slice count due to use of real FFs and instead of SRLs  en=off  latency=1  dbl_ovrd=off  reg_retiming=off  block_type=delay
      settings: xl_area=[0, 0, 0, 0, 0, 0, 0]
  Inverter : xbsIndex_r4/Inverter  en=off  latency=0  dbl_ovrd=off  block_type=inv
      settings: xl_area=[0, 0, 0, 0, 0, 0, 0]
  edge_op : xbsIndex_r4/Logical  logical_function=NOR  inputs=2  en=off  latency=0  precision=Full  arith_type=Unsigned  n_bits=8  bin_pt=2  align_bp=on  dbl_ovrd=off  block_type=logical
      settings: xl_area=[0, 0, 0, 0, 0, 0, 0]
  out : Outport
  wires:
  Inverter/1 -> edge_op/1
  edge_op/1 -> out/1
  in/1 -> Inverter/1, Delay/1
  Delay/1 -> edge_op/2

== system l64_dev/tenge/header/edge_detect10 ==
  in : Inport
  Delay : xbsIndex_r4/Delay  rst=off  infoeditControl=Selection of Reset will increase slice count due to use of real FFs and instead of SRLs  en=off  latency=1  dbl_ovrd=off  reg_retiming=off  block_type=delay
      settings: xl_area=[0, 0, 0, 0, 0, 0, 0]
  Inverter : xbsIndex_r4/Inverter  en=off  latency=0  dbl_ovrd=off  block_type=inv
      settings: xl_area=[0, 0, 0, 0, 0, 0, 0]
  edge_op : xbsIndex_r4/Logical  logical_function=NOR  inputs=2  en=off  latency=0  precision=Full  arith_type=Unsigned  n_bits=8  bin_pt=2  align_bp=on  dbl_ovrd=off  block_type=logical
      settings: xl_area=[0, 0, 0, 0, 0, 0, 0]
  out : Outport
  wires:
  Inverter/1 -> edge_op/1
  edge_op/1 -> out/1
  in/1 -> Inverter/1, Delay/1
  Delay/1 -> edge_op/2

== system l64_dev/tenge/header/edge_detect11 ==
  in : Inport
  Delay : xbsIndex_r4/Delay  rst=off  infoeditControl=Selection of Reset will increase slice count due to use of real FFs and instead of SRLs  en=off  latency=1  dbl_ovrd=off  reg_retiming=off  block_type=delay
      settings: xl_area=[0, 0, 0, 0, 0, 0, 0]
  Inverter : xbsIndex_r4/Inverter  en=off  latency=0  dbl_ovrd=off  block_type=inv
      settings: xl_area=[0, 0, 0, 0, 0, 0, 0]
  edge_op : xbsIndex_r4/Logical  logical_function=NOR  inputs=2  en=off  latency=0  precision=Full  arith_type=Unsigned  n_bits=8  bin_pt=2  align_bp=on  dbl_ovrd=off  block_type=logical
      settings: xl_area=[0, 0, 0, 0, 0, 0, 0]
  out : Outport
  wires:
  Inverter/1 -> edge_op/1
  edge_op/1 -> out/1
  in/1 -> Inverter/1, Delay/1
  Delay/1 -> edge_op/2

== system l64_dev/tenge/header/edge_detect14 ==
  in : Inport
  Delay : xbsIndex_r4/Delay  rst=off  infoeditControl=Selection of Reset will increase slice count due to use of real FFs and instead of SRLs  en=off  latency=1  dbl_ovrd=off  reg_retiming=off  block_type=delay
      settings: xl_area=[0, 0, 0, 0, 0, 0, 0]
  Inverter : xbsIndex_r4/Inverter  en=off  latency=0  dbl_ovrd=off  block_type=inv
      settings: xl_area=[0, 0, 0, 0, 0, 0, 0]
  edge_op : xbsIndex_r4/Logical  logical_function=NOR  inputs=2  en=off  latency=0  precision=Full  arith_type=Unsigned  n_bits=8  bin_pt=2  align_bp=on  dbl_ovrd=off  block_type=logical
      settings: xl_area=[0, 0, 0, 0, 0, 0, 0]
  out : Outport
  wires:
  Inverter/1 -> edge_op/1
  edge_op/1 -> out/1
  in/1 -> Inverter/1, Delay/1
  Delay/1 -> edge_op/2

== system l64_dev/tenge/header/edge_detect15 ==
  in : Inport
  Delay : xbsIndex_r4/Delay  rst=off  infoeditControl=Selection of Reset will increase slice count due to use of real FFs and instead of SRLs  en=off  latency=1  dbl_ovrd=off  reg_retiming=off  block_type=delay
      settings: xl_area=[0, 0, 0, 0, 0, 0, 0]
  Inverter : xbsIndex_r4/Inverter  en=off  latency=0  dbl_ovrd=off  block_type=inv
      settings: xl_area=[0, 0, 0, 0, 0, 0, 0]
  edge_op : xbsIndex_r4/Logical  logical_function=NOR  inputs=2  en=off  latency=0  precision=Full  arith_type=Unsigned  n_bits=8  bin_pt=2  align_bp=on  dbl_ovrd=off  block_type=logical
      settings: xl_area=[0, 0, 0, 0, 0, 0, 0]
  out : Outport
  wires:
  Inverter/1 -> edge_op/1
  edge_op/1 -> out/1
  in/1 -> Inverter/1, Delay/1
  Delay/1 -> edge_op/2

== system l64_dev/tenge/header/edge_detect16 ==
  in : Inport
  Delay : xbsIndex_r4/Delay  rst=off  infoeditControl=Selection of Reset will increase slice count due to use of real FFs and instead of SRLs  en=off  latency=1  dbl_ovrd=off  reg_retiming=off  block_type=delay
      settings: xl_area=[0, 0, 0, 0, 0, 0, 0]
  Inverter : xbsIndex_r4/Inverter  en=off  latency=0  dbl_ovrd=off  block_type=inv
      settings: xl_area=[0, 0, 0, 0, 0, 0, 0]
  edge_op : xbsIndex_r4/Logical  logical_function=NOR  inputs=2  en=off  latency=0  precision=Full  arith_type=Unsigned  n_bits=8  bin_pt=2  align_bp=on  dbl_ovrd=off  block_type=logical
      settings: xl_area=[0, 0, 0, 0, 0, 0, 0]
  out : Outport
  wires:
  Inverter/1 -> edge_op/1
  edge_op/1 -> out/1
  in/1 -> Inverter/1, Delay/1
  Delay/1 -> edge_op/2

== system l64_dev/tenge/header/edge_detect17 ==
  in : Inport
  Delay : xbsIndex_r4/Delay  rst=off  infoeditControl=Selection of Reset will increase slice count due to use of real FFs and instead of SRLs  en=off  latency=1  dbl_ovrd=off  reg_retiming=off  block_type=delay
      settings: xl_area=[0, 0, 0, 0, 0, 0, 0]
  Inverter : xbsIndex_r4/Inverter  en=off  latency=0  dbl_ovrd=off  block_type=inv
      settings: xl_area=[0, 0, 0, 0, 0, 0, 0]
  edge_op : xbsIndex_r4/Logical  logical_function=NOR  inputs=2  en=off  latency=0  precision=Full  arith_type=Unsigned  n_bits=8  bin_pt=2  align_bp=on  dbl_ovrd=off  block_type=logical
      settings: xl_area=[0, 0, 0, 0, 0, 0, 0]
  out : Outport
  wires:
  Inverter/1 -> edge_op/1
  edge_op/1 -> out/1
  in/1 -> Inverter/1, Delay/1
  Delay/1 -> edge_op/2

== system l64_dev/tenge/header/edge_detect2 ==
  in : Inport
  Delay : xbsIndex_r4/Delay  rst=off  infoeditControl=Selection of Reset will increase slice count due to use of real FFs and instead of SRLs  en=off  latency=1  dbl_ovrd=off  reg_retiming=off  block_type=delay
      settings: xl_area=[0, 0, 0, 0, 0, 0, 0]
  Inverter : xbsIndex_r4/Inverter  en=off  latency=0  dbl_ovrd=off  block_type=inv
      settings: xl_area=[0, 0, 0, 0, 0, 0, 0]
  edge_op : xbsIndex_r4/Logical  logical_function=NOR  inputs=2  en=off  latency=0  precision=Full  arith_type=Unsigned  n_bits=8  bin_pt=2  align_bp=on  dbl_ovrd=off  block_type=logical
      settings: xl_area=[0, 0, 0, 0, 0, 0, 0]
  out : Outport
  wires:
  Inverter/1 -> edge_op/1
  edge_op/1 -> out/1
  in/1 -> Inverter/1, Delay/1
  Delay/1 -> edge_op/2

== system l64_dev/tenge/header/edge_detect3 ==
  in : Inport
  Delay : xbsIndex_r4/Delay  rst=off  infoeditControl=Selection of Reset will increase slice count due to use of real FFs and instead of SRLs  en=off  latency=1  dbl_ovrd=off  reg_retiming=off  block_type=delay
      settings: xl_area=[0, 0, 0, 0, 0, 0, 0]
  Inverter : xbsIndex_r4/Inverter  en=off  latency=0  dbl_ovrd=off  block_type=inv
      settings: xl_area=[0, 0, 0, 0, 0, 0, 0]
  edge_op : xbsIndex_r4/Logical  logical_function=NOR  inputs=2  en=off  latency=0  precision=Full  arith_type=Unsigned  n_bits=8  bin_pt=2  align_bp=on  dbl_ovrd=off  block_type=logical
      settings: xl_area=[0, 0, 0, 0, 0, 0, 0]
  out : Outport
  wires:
  Inverter/1 -> edge_op/1
  edge_op/1 -> out/1
  in/1 -> Inverter/1, Delay/1
  Delay/1 -> edge_op/2

== system l64_dev/tenge/header/edge_detect4 ==
  in : Inport
  Delay : xbsIndex_r4/Delay  rst=off  infoeditControl=Selection of Reset will increase slice count due to use of real FFs and instead of SRLs  en=off  latency=1  dbl_ovrd=off  reg_retiming=off  block_type=delay
      settings: xl_area=[0, 0, 0, 0, 0, 0, 0]
  Inverter : xbsIndex_r4/Inverter  en=off  latency=0  dbl_ovrd=off  block_type=inv
      settings: xl_area=[0, 0, 0, 0, 0, 0, 0]
  edge_op : xbsIndex_r4/Logical  logical_function=NOR  inputs=2  en=off  latency=0  precision=Full  arith_type=Unsigned  n_bits=8  bin_pt=2  align_bp=on  dbl_ovrd=off  block_type=logical
      settings: xl_area=[0, 0, 0, 0, 0, 0, 0]
  out : Outport
  wires:
  Inverter/1 -> edge_op/1
  edge_op/1 -> out/1
  in/1 -> Inverter/1, Delay/1
  Delay/1 -> edge_op/2

== system l64_dev/tenge/header/edge_detect9 ==
  in : Inport
  Delay : xbsIndex_r4/Delay  rst=off  infoeditControl=Selection of Reset will increase slice count due to use of real FFs and instead of SRLs  en=off  latency=1  dbl_ovrd=off  reg_retiming=off  block_type=delay
      settings: xl_area=[0, 0, 0, 0, 0, 0, 0]
  Inverter : xbsIndex_r4/Inverter  en=off  latency=0  dbl_ovrd=off  block_type=inv
      settings: xl_area=[0, 0, 0, 0, 0, 0, 0]
  edge_op : xbsIndex_r4/Logical  logical_function=NOR  inputs=2  en=off  latency=0  precision=Full  arith_type=Unsigned  n_bits=8  bin_pt=2  align_bp=on  dbl_ovrd=off  block_type=logical
      settings: xl_area=[0, 0, 0, 0, 0, 0, 0]
  out : Outport
  wires:
  Inverter/1 -> edge_op/1
  edge_op/1 -> out/1
  in/1 -> Inverter/1, Delay/1
  Delay/1 -> edge_op/2
